simulink subsystem "Magnetometer"  (R2023a)
settings: Solver=VariableStepAuto  StartTime=0.0  StopTime=10.0  RelTol=1e-3
libraries: mbedblockslib x2
settings Model: Creator=JesseJabezArendse  LastModifiedBy=JesseJabezArendse

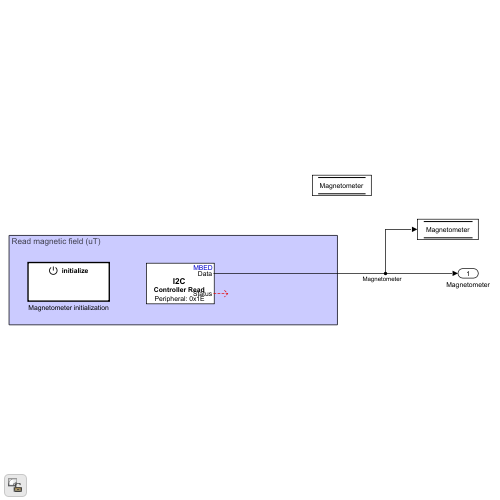
[thumbnail: Simulink's stored preview of the top-level diagram]
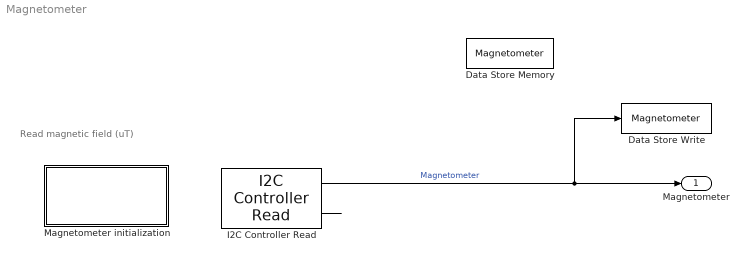
== system Magnetometer ==
  note: Read magnetic field (uT)
  Data Store Memory : DataStoreMemory  DataStoreName=Magnetometer  WriteAfterWriteMsg=warning  ShowAdditionalParam=off  OutDataTypeStr=int16  Dimensions=3
  Data Store Write : DataStoreWrite  DataStoreName=Magnetometer  IndexOptions=Index vector (dialog)  Indices=1  OutputSizes=1
  I2C Controller Read : mbedblockslib/I2C Controller Read  I2CModule=0  Mode=Master  SlaveAddress=0x1E  SlaveByteOrder=LittleEndian  Direction=Receiver  RegisterAddressMode=on  RegisterAddress=0x68  SlaveDataType=int16  DataLength=3  NoAck=off  RepeatedStart=off  OutputStatus=on  SampleTime=0.01
      settings: LibrarySourceBlock=stmnucleorootlib/Common/I2C Controller Read
  Magnetometer initialization : Subsystem  TreatAsAtomicUnit=on
  Magnetometer : Outport
  wires:
  I2C Controller Read/1 -> Data Store Write/1, Magnetometer/1  "Magnetometer"
  I2C Controller Read/2 -> ?

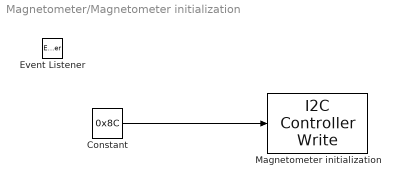
== system Magnetometer/Magnetometer initialization ==
  Constant : Constant  Value=0x8C  OutDataTypeStr=uint8
  Event Listener : EventListener  DisableCoverage=on  EventName=reset
  Magnetometer initialization : mbedblockslib/I2C Controller Write  I2CModule=0  Mode=Master  SlaveAddress=0x1E  SlaveByteOrder=BigEndian  Direction=Transmitter  RegisterAddressMode=on  RegisterAddress=0x60  SlaveDataType=uint8  DataLength=2  NoAck=off  RepeatedStart=off  OutputStatus=on
      settings: LibrarySourceBlock=stmnucleorootlib/Common/I2C Controller Write
  wires:
  Constant/1 -> Magnetometer initialization/1
